simulink model "text28"  (R2014a)
settings: Solver=FixedStepDiscrete  StartTime=0.0  StopTime=10.0  FixedStep=0.0005  RelTol=1e-3
libraries: simulink x70, ec55xxlib x61
(part 2 of 3)

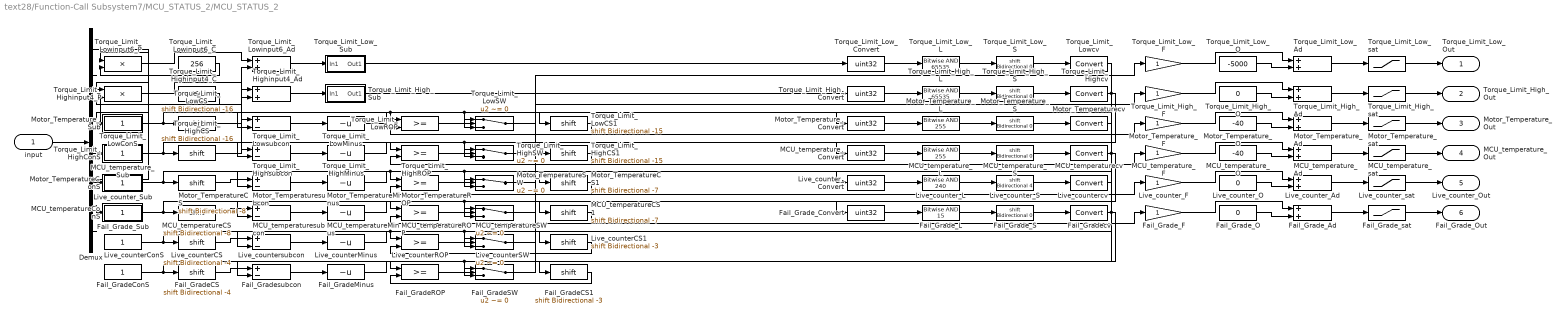
== system text28/Function-Call Subsystem7/MCU_STATUS_2/MCU_STATUS_2 ==
  input : Inport
  Demux : Demux  Outputs=8
  Fail_GradeCS : ArithShift  BitShiftNumber=-4
  Fail_GradeCS1 : ArithShift  BitShiftNumber=-3
  Fail_GradeConS : Constant  OutDataTypeStr=single
  Fail_GradeMinus : UnaryMinus
  Fail_GradeROP : RelationalOperator  OutDataTypeStr=boolean
  Fail_GradeSW : Switch  Criteria=u2 ~= 0
  Fail_Grade_Ad : Sum
  Fail_Grade_Convert : DataTypeConversion  OutDataTypeStr=uint32
  Fail_Grade_F : Gain
  Fail_Grade_L : simulink/Logic and Bit Operations/Bitwise Operator  logicop=AND  UseBitMask=on  BitMask=15  BitMaskRealWorld=Stored Integer
  Fail_Grade_O : Constant  Value=0  OutDataTypeStr=single
  Fail_Grade_S : ArithShift
  Fail_Grade_Sub : Subsystem
  Fail_Grade_sat : Saturate  UpperLimit=4  LowerLimit=0
  Fail_Gradecv : DataTypeConversion
  Fail_Gradesubcon : Sum  Inputs=+-
  Live_counterCS : ArithShift  BitShiftNumber=-4
  Live_counterCS1 : ArithShift  BitShiftNumber=-3
  Live_counterConS : Constant  OutDataTypeStr=single
  Live_counterMinus : UnaryMinus
  Live_counterROP : RelationalOperator  OutDataTypeStr=boolean
  Live_counterSW : Switch  Criteria=u2 ~= 0
  Live_counter_Ad : Sum
  Live_counter_Convert : DataTypeConversion  OutDataTypeStr=uint32
  Live_counter_F : Gain
  Live_counter_L : simulink/Logic and Bit Operations/Bitwise Operator  logicop=AND  UseBitMask=on  BitMask=240  BitMaskRealWorld=Stored Integer
  Live_counter_O : Constant  Value=0  OutDataTypeStr=single
  Live_counter_S : ArithShift  BitShiftNumber=4
  Live_counter_Sub : Subsystem
  Live_counter_sat : Saturate  UpperLimit=15  LowerLimit=0
  Live_countercv : DataTypeConversion
  Live_countersubcon : Sum  Inputs=+-
  MCU_temperatureCS : ArithShift  BitShiftNumber=-8
  MCU_temperatureCS1 : ArithShift  BitShiftNumber=-7
  MCU_temperatureConS : Constant  OutDataTypeStr=single
  MCU_temperatureMinus : UnaryMinus
  MCU_temperatureROP : RelationalOperator  OutDataTypeStr=boolean
  MCU_temperatureSW : Switch  Criteria=u2 ~= 0
  MCU_temperature_Ad : Sum
  MCU_temperature_Convert : DataTypeConversion  OutDataTypeStr=uint32
  MCU_temperature_F : Gain
  MCU_temperature_L : simulink/Logic and Bit Operations/Bitwise Operator  logicop=AND  UseBitMask=on  BitMask=255  BitMaskRealWorld=Stored Integer
  MCU_temperature_O : Constant  Value=-40  OutDataTypeStr=single
  MCU_temperature_S : ArithShift
  MCU_temperature_Sub : Subsystem
  MCU_temperature_sat : Saturate  UpperLimit=215  LowerLimit=-40
  MCU_temperaturecv : DataTypeConversion
  MCU_temperaturesubcon : Sum  Inputs=+-
  Motor_TemperatureCS : ArithShift  BitShiftNumber=-8
  Motor_TemperatureCS1 : ArithShift  BitShiftNumber=-7
  Motor_TemperatureConS : Constant  OutDataTypeStr=single
  Motor_TemperatureMinus : UnaryMinus
  Motor_TemperatureROP : RelationalOperator  OutDataTypeStr=boolean
  Motor_TemperatureSW : Switch  Criteria=u2 ~= 0
  Motor_Temperature_Ad : Sum
  Motor_Temperature_Convert : DataTypeConversion  OutDataTypeStr=uint32
  Motor_Temperature_F : Gain
  Motor_Temperature_L : simulink/Logic and Bit Operations/Bitwise Operator  logicop=AND  UseBitMask=on  BitMask=255  BitMaskRealWorld=Stored Integer
  Motor_Temperature_O : Constant  Value=-40  OutDataTypeStr=single
  Motor_Temperature_S : ArithShift
  Motor_Temperature_Sub : Subsystem
  Motor_Temperature_sat : Saturate  UpperLimit=215  LowerLimit=-40
  Motor_Temperaturecv : DataTypeConversion
  Motor_Temperaturesubcon : Sum  Inputs=+-
  Torque_Limit_HighCS : ArithShift  BitShiftNumber=-16
  Torque_Limit_HighCS1 : ArithShift  BitShiftNumber=-15
  Torque_Limit_HighConS : Constant  OutDataTypeStr=single
  Torque_Limit_HighMinus : UnaryMinus
  Torque_Limit_HighROP : RelationalOperator  OutDataTypeStr=boolean
  Torque_Limit_HighSW : Switch  Criteria=u2 ~= 0
  Torque_Limit_High_Ad : Sum
  Torque_Limit_High_Convert : DataTypeConversion  OutDataTypeStr=uint32
  Torque_Limit_High_F : Gain
  Torque_Limit_High_L : simulink/Logic and Bit Operations/Bitwise Operator  logicop=AND  UseBitMask=on  BitMask=65535  BitMaskRealWorld=Stored Integer
  Torque_Limit_High_O : Constant  Value=0  OutDataTypeStr=single
  Torque_Limit_High_S : ArithShift
  Torque_Limit_High_Sub : Subsystem
  Torque_Limit_High_sat : Saturate  UpperLimit=5000  LowerLimit=0
  Torque_Limit_Highcv : DataTypeConversion
  Torque_Limit_Highinput4_Ad : Sum
  Torque_Limit_Highinput4_C : Constant  Value=256
  Torque_Limit_Highinput4_P : Product
  Torque_Limit_Highsubcon : Sum  Inputs=+-
  Torque_Limit_LowCS : ArithShift  BitShiftNumber=-16
  Torque_Limit_LowCS1 : ArithShift  BitShiftNumber=-15
  Torque_Limit_LowConS : Constant  OutDataTypeStr=single
  Torque_Limit_LowMinus : UnaryMinus
  Torque_Limit_LowROP : RelationalOperator  OutDataTypeStr=boolean
  Torque_Limit_LowSW : Switch  Criteria=u2 ~= 0
  Torque_Limit_Low_Ad : Sum
  Torque_Limit_Low_Convert : DataTypeConversion  OutDataTypeStr=uint32
  Torque_Limit_Low_F : Gain
  Torque_Limit_Low_L : simulink/Logic and Bit Operations/Bitwise Operator  logicop=AND  UseBitMask=on  BitMask=65535  BitMaskRealWorld=Stored Integer
  Torque_Limit_Low_O : Constant  Value=-5000  OutDataTypeStr=single
  Torque_Limit_Low_S : ArithShift
  Torque_Limit_Low_Sub : Subsystem
  Torque_Limit_Low_sat : Saturate  UpperLimit=0  LowerLimit=-5000
  Torque_Limit_Lowcv : DataTypeConversion
  Torque_Limit_Lowinput6_Ad : Sum
  Torque_Limit_Lowinput6_C : Constant  Value=256
  Torque_Limit_Lowinput6_P : Product
  Torque_Limit_Lowsubcon : Sum  Inputs=+-
  Torque_Limit_Low_Out : Outport
  Torque_Limit_High_Out : Outport  Port=2
  Motor_Temperature_Out : Outport  Port=3
  MCU_temperature_Out : Outport  Port=4
  Live_counter_Out : Outport  Port=5
  Fail_Grade_Out : Outport  Port=6
  wires:
  Torque_Limit_Low_F/1 -> Torque_Limit_Low_Ad/1
  Torque_Limit_Low_O/1 -> Torque_Limit_Low_Ad/2
  Torque_Limit_Low_Ad/1 -> Torque_Limit_Low_sat/1
  Torque_Limit_Low_sat/1 -> Torque_Limit_Low_Out/1
  Demux/6 -> Torque_Limit_Lowinput6_P/1
  Torque_Limit_Lowinput6_C/1 -> Torque_Limit_Lowinput6_P/2
  Torque_Limit_Lowinput6_P/1 -> Torque_Limit_Lowinput6_Ad/1
  Demux/5 -> Torque_Limit_Lowinput6_Ad/2
  Torque_Limit_Lowinput6_Ad/1 -> Torque_Limit_Low_Sub/1(In1)
  Torque_Limit_Low_Sub/1(Out1) -> Torque_Limit_Low_Convert/1
  Torque_Limit_Low_Convert/1 -> Torque_Limit_Low_L/1
  Torque_Limit_Low_L/1 -> Torque_Limit_Low_S/1
  Torque_Limit_Low_S/1 -> Torque_Limit_Lowcv/1
  Torque_Limit_Lowcv/1 -> Torque_Limit_LowROP/1, Torque_Limit_Lowsubcon/2, Torque_Limit_LowSW/3
  Torque_Limit_LowConS/1 -> Torque_Limit_LowCS/1, Torque_Limit_LowCS1/1
  Torque_Limit_LowCS1/1 -> Torque_Limit_LowROP/2
  Torque_Limit_LowCS/1 -> Torque_Limit_Lowsubcon/1
  Torque_Limit_Lowsubcon/1 -> Torque_Limit_LowMinus/1
  Torque_Limit_LowMinus/1 -> Torque_Limit_LowSW/1
  Torque_Limit_LowSW/1 -> Torque_Limit_Low_F/1
  Torque_Limit_LowROP/1 -> Torque_Limit_LowSW/2
  Torque_Limit_High_F/1 -> Torque_Limit_High_Ad/1
  Torque_Limit_High_O/1 -> Torque_Limit_High_Ad/2
  Torque_Limit_High_Ad/1 -> Torque_Limit_High_sat/1
  Torque_Limit_High_sat/1 -> Torque_Limit_High_Out/1
  Demux/4 -> Torque_Limit_Highinput4_P/1
  Torque_Limit_Highinput4_C/1 -> Torque_Limit_Highinput4_P/2
  Torque_Limit_Highinput4_P/1 -> Torque_Limit_Highinput4_Ad/1
  Demux/3 -> Torque_Limit_Highinput4_Ad/2
  Torque_Limit_Highinput4_Ad/1 -> Torque_Limit_High_Sub/1(In1)
  Torque_Limit_High_Sub/1(Out1) -> Torque_Limit_High_Convert/1
  Torque_Limit_High_Convert/1 -> Torque_Limit_High_L/1
  Torque_Limit_High_L/1 -> Torque_Limit_High_S/1
  Torque_Limit_High_S/1 -> Torque_Limit_Highcv/1
  Torque_Limit_Highcv/1 -> Torque_Limit_Highsubcon/2, Torque_Limit_HighSW/3, Torque_Limit_HighROP/1
  Torque_Limit_HighConS/1 -> Torque_Limit_HighCS/1, Torque_Limit_HighCS1/1
  Torque_Limit_HighCS1/1 -> Torque_Limit_HighROP/2
  Torque_Limit_HighCS/1 -> Torque_Limit_Highsubcon/1
  Torque_Limit_Highsubcon/1 -> Torque_Limit_HighMinus/1
  Torque_Limit_HighMinus/1 -> Torque_Limit_HighSW/1
  Torque_Limit_HighSW/1 -> Torque_Limit_High_F/1
  Torque_Limit_HighROP/1 -> Torque_Limit_HighSW/2
  Motor_Temperature_F/1 -> Motor_Temperature_Ad/1
  Motor_Temperature_O/1 -> Motor_Temperature_Ad/2
  Motor_Temperature_Ad/1 -> Motor_Temperature_sat/1
  Motor_Temperature_sat/1 -> Motor_Temperature_Out/1
  Demux/1 -> Motor_Temperature_Sub/1(In1)
  Motor_Temperature_Sub/1(Out1) -> Motor_Temperature_Convert/1
  Motor_Temperature_Convert/1 -> Motor_Temperature_L/1
  Motor_Temperature_L/1 -> Motor_Temperature_S/1
  Motor_Temperature_S/1 -> Motor_Temperaturecv/1
  Motor_Temperaturecv/1 -> Motor_TemperatureROP/1, Motor_Temperaturesubcon/2, Motor_TemperatureSW/3
  Motor_TemperatureConS/1 -> Motor_TemperatureCS/1, Motor_TemperatureCS1/1
  Motor_TemperatureCS1/1 -> Motor_TemperatureROP/2
  Motor_TemperatureCS/1 -> Motor_Temperaturesubcon/1
  Motor_Temperaturesubcon/1 -> Motor_TemperatureMinus/1
  Motor_TemperatureMinus/1 -> Motor_TemperatureSW/1
  Motor_TemperatureSW/1 -> Motor_Temperature_F/1
  Motor_TemperatureROP/1 -> Motor_TemperatureSW/2
  MCU_temperature_F/1 -> MCU_temperature_Ad/1
  MCU_temperature_O/1 -> MCU_temperature_Ad/2
  MCU_temperature_Ad/1 -> MCU_temperature_sat/1
  MCU_temperature_sat/1 -> MCU_temperature_Out/1
  Demux/2 -> MCU_temperature_Sub/1(In1)
  MCU_temperature_Sub/1(Out1) -> MCU_temperature_Convert/1
  MCU_temperature_Convert/1 -> MCU_temperature_L/1
  MCU_temperature_L/1 -> MCU_temperature_S/1
  MCU_temperature_S/1 -> MCU_temperaturecv/1
  MCU_temperaturecv/1 -> MCU_temperaturesubcon/2, MCU_temperatureSW/3, MCU_temperatureROP/1
  MCU_temperatureConS/1 -> MCU_temperatureCS/1, MCU_temperatureCS1/1
  MCU_temperatureCS1/1 -> MCU_temperatureROP/2
  MCU_temperatureCS/1 -> MCU_temperaturesubcon/1
  MCU_temperaturesubcon/1 -> MCU_temperatureMinus/1
  MCU_temperatureMinus/1 -> MCU_temperatureSW/1
  MCU_temperatureSW/1 -> MCU_temperature_F/1
  MCU_temperatureROP/1 -> MCU_temperatureSW/2
  Live_counter_F/1 -> Live_counter_Ad/1
  Live_counter_O/1 -> Live_counter_Ad/2
  Live_counter_Ad/1 -> Live_counter_sat/1
  Live_counter_sat/1 -> Live_counter_Out/1
  Demux/8 -> Live_counter_Sub/1(In1)
  Live_counter_Sub/1(Out1) -> Live_counter_Convert/1
  Live_counter_Convert/1 -> Live_counter_L/1
  Live_counter_L/1 -> Live_counter_S/1
  Live_counter_S/1 -> Live_countercv/1
  Live_countercv/1 -> Live_counterROP/1, Live_countersubcon/2, Live_counterSW/3
  Live_counterConS/1 -> Live_counterCS/1, Live_counterCS1/1
  Live_counterCS1/1 -> Live_counterROP/2
  Live_counterCS/1 -> Live_countersubcon/1
  Live_countersubcon/1 -> Live_counterMinus/1
  Live_counterMinus/1 -> Live_counterSW/1
  Live_counterSW/1 -> Live_counter_F/1
  Live_counterROP/1 -> Live_counterSW/2
  Fail_Grade_F/1 -> Fail_Grade_Ad/1
  Fail_Grade_O/1 -> Fail_Grade_Ad/2
  Fail_Grade_Ad/1 -> Fail_Grade_sat/1
  Fail_Grade_sat/1 -> Fail_Grade_Out/1
  Demux/7 -> Fail_Grade_Sub/1(In1)
  Fail_Grade_Sub/1(Out1) -> Fail_Grade_Convert/1
  Fail_Grade_Convert/1 -> Fail_Grade_L/1
  Fail_Grade_L/1 -> Fail_Grade_S/1
  Fail_Grade_S/1 -> Fail_Gradecv/1
  Fail_Gradecv/1 -> Fail_Gradesubcon/2, Fail_GradeSW/3, Fail_GradeROP/1
  Fail_GradeConS/1 -> Fail_GradeCS/1, Fail_GradeCS1/1
  Fail_GradeCS1/1 -> Fail_GradeROP/2
  Fail_GradeCS/1 -> Fail_Gradesubcon/1
  Fail_Gradesubcon/1 -> Fail_GradeMinus/1
  Fail_GradeMinus/1 -> Fail_GradeSW/1
  Fail_GradeSW/1 -> Fail_Grade_F/1
  Fail_GradeROP/1 -> Fail_GradeSW/2
  input/1 -> Demux/1

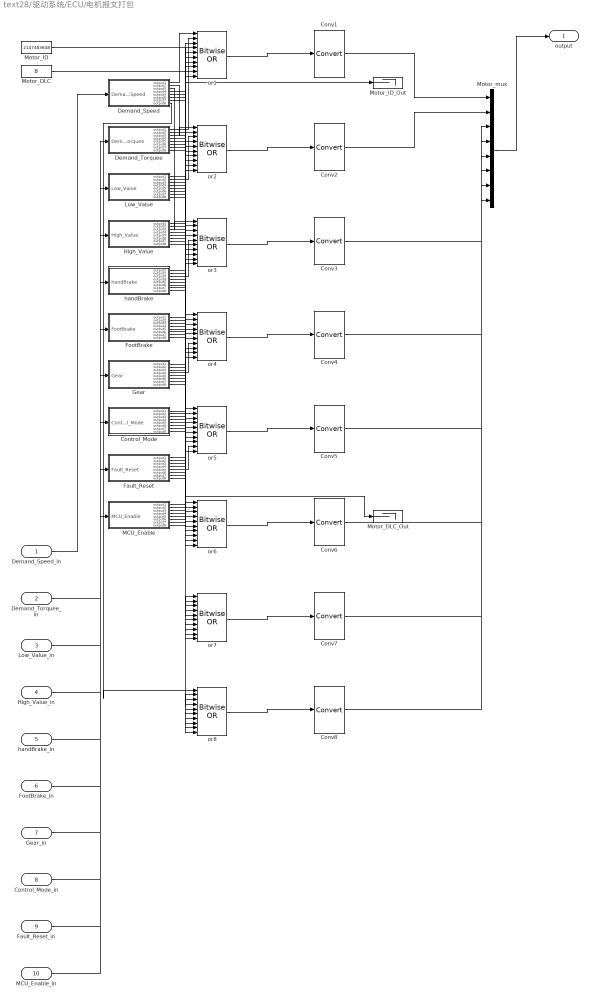
== system text28/驱动系统/ECU/电机报文打包 ==
  Demand_Speed_in : Inport
  Demand_Torquee_in : Inport  Port=2
  Low_Value_in : Inport  Port=3
  High_Value_in : Inport  Port=4
  handBrake_in : Inport  Port=5
  FootBrake_in : Inport  Port=6
  Gear_in : Inport  Port=7
  Control_Mode_in : Inport  Port=8
  Fault_Reset_in : Inport  Port=9
  MCU_Enable_in : Inport  Port=10
  Control_Mode : Subsystem
  Conv{1..8} (8 alike) : DataTypeConversion
  Demand_Speed : Subsystem
  Demand_Torquee : Subsystem
  Fault_Reset : Subsystem
  FootBrake : Subsystem
  Gear : Subsystem
  High_Value : Subsystem
  Low_Value : Subsystem
  MCU_Enable : Subsystem
  Motor_DLC : Constant  Value=8  OutDataTypeStr=uint8
  Motor_DLC_Out : Terminator
  Motor_ID : Constant  Value=2147483648  OutDataTypeStr=single
  Motor_ID_Out : Terminator
  Motor_mux : Mux  Inputs=8
  handBrake : Subsystem
  or{1..8} (8 alike) : simulink/Logic and Bit Operations/Bitwise Operator  logicop=OR  UseBitMask=off  NumInputPorts=10  BitMask=bin2dec('11011001')  BitMaskRealWorld=Stored Integer
  output : Outport
  wires:
  MCU_Enable_in/1 -> MCU_Enable/1(MCU_Enable)
  Fault_Reset_in/1 -> Fault_Reset/1(Fault_Reset)
  Control_Mode_in/1 -> Control_Mode/1(Control_Mode)
  Gear_in/1 -> Gear/1(Gear)
  FootBrake_in/1 -> FootBrake/1(FootBrake)
  handBrake_in/1 -> handBrake/1(handBrake)
  High_Value_in/1 -> High_Value/1(High_Value)
  Low_Value_in/1 -> Low_Value/1(Low_Value)
  Demand_Torquee_in/1 -> Demand_Torquee/1(Demand_Torquee)
  Demand_Speed_in/1 -> Demand_Speed/1(Demand_Speed)
  Motor_DLC/1 -> Motor_DLC_Out/1
  Motor_ID/1 -> Motor_ID_Out/1
  Conv8/1 -> Motor_mux/8
  or8/1 -> Conv8/1
  Conv7/1 -> Motor_mux/7
  or7/1 -> Conv7/1
  Conv6/1 -> Motor_mux/6
  or6/1 -> Conv6/1
  Conv5/1 -> Motor_mux/5
  or5/1 -> Conv5/1
  Conv4/1 -> Motor_mux/4
  or4/1 -> Conv4/1
  Conv3/1 -> Motor_mux/3
  or3/1 -> Conv3/1
  Conv2/1 -> Motor_mux/2
  or2/1 -> Conv2/1
  Conv1/1 -> Motor_mux/1
  or1/1 -> Conv1/1
  MCU_Enable/8(output8) -> or8/10
  MCU_Enable/7(output7) -> or7/10
  MCU_Enable/6(output6) -> or6/10
  MCU_Enable/5(output5) -> or5/10
  MCU_Enable/4(output4) -> or4/10
  MCU_Enable/3(output3) -> or3/10
  MCU_Enable/2(output2) -> or2/10
  MCU_Enable/1(output1) -> or1/10
  Fault_Reset/8(output8) -> or8/9
  Fault_Reset/7(output7) -> or7/9
  Fault_Reset/6(output6) -> or6/9
  Fault_Reset/5(output5) -> or5/9
  Fault_Reset/4(output4) -> or4/9
  Fault_Reset/3(output3) -> or3/9
  Fault_Reset/2(output2) -> or2/9
  Fault_Reset/1(output1) -> or1/9
  Control_Mode/8(output8) -> or8/8
  Control_Mode/7(output7) -> or7/8
  Control_Mode/6(output6) -> or6/8
  Control_Mode/5(output5) -> or5/8
  Control_Mode/4(output4) -> or4/8
  Control_Mode/3(output3) -> or3/8
  Control_Mode/2(output2) -> or2/8
  Control_Mode/1(output1) -> or1/8
  Gear/8(output8) -> or8/7
  Gear/7(output7) -> or7/7
  Gear/6(output6) -> or6/7
  Gear/5(output5) -> or5/7
  Gear/4(output4) -> or4/7
  Gear/3(output3) -> or3/7
  Gear/2(output2) -> or2/7
  Gear/1(output1) -> or1/7
  FootBrake/8(output8) -> or8/6
  FootBrake/7(output7) -> or7/6
  FootBrake/6(output6) -> or6/6
  FootBrake/5(output5) -> or5/6
  FootBrake/4(output4) -> or4/6
  FootBrake/3(output3) -> or3/6
  FootBrake/2(output2) -> or2/6
  FootBrake/1(output1) -> or1/6
  handBrake/8(output8) -> or8/5
  handBrake/7(output7) -> or7/5
  handBrake/6(output6) -> or6/5
  handBrake/5(output5) -> or5/5
  handBrake/4(output4) -> or4/5
  handBrake/3(output3) -> or3/5
  handBrake/2(output2) -> or2/5
  handBrake/1(output1) -> or1/5
  High_Value/8(output8) -> or8/4
  High_Value/7(output7) -> or7/4
  High_Value/6(output6) -> or6/4
  High_Value/5(output5) -> or5/4
  High_Value/4(output4) -> or4/4
  High_Value/3(output3) -> or3/4
  High_Value/2(output2) -> or2/4
  High_Value/1(output1) -> or1/4
  Low_Value/8(output8) -> or8/3
  Low_Value/7(output7) -> or7/3
  Low_Value/6(output6) -> or6/3
  Low_Value/5(output5) -> or5/3
  Low_Value/4(output4) -> or4/3
  Low_Value/3(output3) -> or3/3
  Low_Value/2(output2) -> or2/3
  Low_Value/1(output1) -> or1/3
  Demand_Torquee/8(output8) -> or8/2
  Demand_Torquee/7(output7) -> or7/2
  Demand_Torquee/6(output6) -> or6/2
  Demand_Torquee/5(output5) -> or5/2
  Demand_Torquee/4(output4) -> or4/2
  Demand_Torquee/3(output3) -> or3/2
  Demand_Torquee/2(output2) -> or2/2
  Demand_Torquee/1(output1) -> or1/2
  Demand_Speed/8(output8) -> or8/1
  Demand_Speed/7(output7) -> or7/1
  Demand_Speed/6(output6) -> or6/1
  Demand_Speed/5(output5) -> or5/1
  Demand_Speed/4(output4) -> or4/1
  Demand_Speed/3(output3) -> or3/1
  Demand_Speed/2(output2) -> or2/1
  Demand_Speed/1(output1) -> or1/1
  Motor_mux/1 -> output/1

== system text28/驱动系统/MCU_CAN发送/安全回路out ==
  CAN ok : Inport
  Data Type Conversion1 : DataTypeConversion  OutDataTypeStr=double
  If : If  IfExpression=u1 < 2
  If Action Subsystem1 : Subsystem  TreatAsAtomicUnit=on
  If Action Subsystem2 : Subsystem  TreatAsAtomicUnit=on
  Merge : Merge
  Out1 : Outport
  wires:
  If/1 -> If Action Subsystem2/Action
  If/2 -> If Action Subsystem1/Action
  If Action Subsystem1/1(Out2) -> Merge/2
  If Action Subsystem2/1(Out1) -> Merge/1
  CAN ok/1 -> Data Type Conversion1/1
  Data Type Conversion1/1 -> If/1
  Merge/1 -> Out1/1

== system text28/驱动系统/驱动逻辑/Drive_AEKF ==
  T_base : Inport
  w_rpm : Inport  Port=2
  Te_raw : Inport  Port=3
  T_base_d : DataTypeConversion  OutDataTypeStr=double  SaturateOnIntegerOverflow=on  RndMeth=Zero
  Te_raw_d : DataTypeConversion  OutDataTypeStr=double  SaturateOnIntegerOverflow=on  RndMeth=Zero
  TorqueDelta : Sum  Inputs=+-  SaturateOnIntegerOverflow=on  InputSameDT=on  OutDataTypeStr=Inherit: Same as first input
  TorqueDeltaSat : Saturate  UpperLimit=25  LowerLimit=-50
  TorquePrev : UnitDelay  SampleTime=-1
  TorqueSum : Sum  SaturateOnIntegerOverflow=on  InputSameDT=on  OutDataTypeStr=Inherit: Same as first input
  aekf_comp : MATLAB Function  TreatAsAtomicUnit=on
  w_rpm_d : DataTypeConversion  OutDataTypeStr=double  SaturateOnIntegerOverflow=on  RndMeth=Zero
  T_opt : Outport
  wires:
  T_base/1 -> T_base_d/1
  w_rpm/1 -> w_rpm_d/1
  Te_raw/1 -> Te_raw_d/1
  T_base_d/1 -> aekf_comp/1(T_base)
  w_rpm_d/1 -> aekf_comp/2(w_rpm)
  Te_raw_d/1 -> aekf_comp/3(Te_raw)
  aekf_comp/1(T_opt) -> TorqueDelta/1
  TorquePrev/1 -> TorqueDelta/2, TorqueSum/1
  TorqueDelta/1 -> TorqueDeltaSat/1
  TorqueDeltaSat/1 -> TorqueSum/2
  TorqueSum/1 -> T_opt/1, TorquePrev/1

== system text28/驱动系统/驱动逻辑/制动与尾灯 ==
  Constant2 : Constant  OutDataTypeStr=uint32  SampleTime=-1
  Data Type Conversion : DataTypeConversion  OutDataTypeStr=uint32
  If : If  IfExpression=u1 > 550 &u1 < 4600
  If Action Subsystem : Subsystem  TreatAsAtomicUnit=on
  If Action Subsystem1 : Subsystem  TreatAsAtomicUnit=on
  If Action Subsystem2 : Subsystem  TreatAsAtomicUnit=on
  If Action Subsystem3 : Subsystem  TreatAsAtomicUnit=on
  If1 : If  IfExpression=u1 > 850 &u1 < 4600
  MeaModule : ec55xxlib/RapidECU_U2/11Calibration/MeaModule  signal=youya1
  MeaModule1 : ec55xxlib/RapidECU_U2/11Calibration/MeaModule  signal=youya2
  MeaModule2 : ec55xxlib/RapidECU_U2/11Calibration/MeaModule  signal=youya3
  Merge1 : Merge
  Merge4 : Merge
  前油压 : ec55xxlib/RapidECU_U2/02AnalogInput/AnalogInput  channel=54: I_AN15_5V  sampletime=-1
  尾灯 : ec55xxlib/RapidECU_U2/06PowerDriverPWM/PowerDriverPWM  channel=115: O_PWM10_HS2A9  sampletime=-1
  油压2 : Outport
  油压1 : Outport  Port=2
  wires:
  If/1 -> If Action Subsystem/Action
  If/2 -> If Action Subsystem1/Action
  If Action Subsystem1/1(Out1) -> Merge4/2
  If Action Subsystem/1(Out1) -> Merge4/1
  Constant2/1 -> 尾灯/1
  Data Type Conversion/1 -> 尾灯/2
  前油压/1 -> MeaModule/1
  Merge4/1 -> MeaModule1/1, Data Type Conversion/1
  If1/1 -> If Action Subsystem2/Action
  If1/2 -> If Action Subsystem3/Action
  If Action Subsystem3/1(Out1) -> Merge1/2
  If Action Subsystem2/1(Out1) -> Merge1/1
  MeaModule/1 -> If1/1, If/1
  Merge1/1 -> MeaModule2/1
  MeaModule2/1 -> 油压2/1
  MeaModule1/1 -> 油压1/1

== system text28/驱动系统/驱动逻辑/制动与待驶 ==
  note: `
  "制动 " : Inport
  Constant : Constant  Value=0  SampleTime=-1
  Constant1 : Constant  SampleTime=-1
  Logical Operator : Logic  AllPortsSameDT=off  OutDataTypeStr=boolean
  MeaModule : ec55xxlib/RapidECU_U2/11Calibration/MeaModule  signal=enable_sign
  MeaModule1 : ec55xxlib/RapidECU_U2/11Calibration/MeaModule  signal=daishi
  MeaModule2 : ec55xxlib/RapidECU_U2/11Calibration/MeaModule  signal=aqhl
  MeaModule3 : ec55xxlib/RapidECU_U2/11Calibration/MeaModule  signal=daishi_chu
  MeaModule4 : ec55xxlib/RapidECU_U2/11Calibration/MeaModule  signal=daishi_fanhui
  MeaModule5 : ec55xxlib/RapidECU_U2/11Calibration/MeaModule  signal=daishi_out
  Product : Product
  Saturation : Saturate  UpperLimit=1  LowerLimit=0
  Sum : Sum  Inputs=|++
  Switch : Switch  Criteria=u2 > Threshold
  SwitchInput : ec55xxlib/RapidECU_U2/01SwitchInput/SwitchInput  channel=44: I_SW11_H  sampletime=-1
  Unit Delay : UnitDelay  SampleTime=-1
  待驶按键 : Subsystem
  待驶激活 : Subsystem
  鸣笛1 : Subsystem
  RES : Outport
  EN : Outport  Port=2
  wires:
  Constant/1 -> Switch/1
  Constant1/1 -> Switch/3
  Switch/1 -> RES/1
  Saturation/1 -> MeaModule/1
  Unit Delay/1 -> MeaModule4/1
  "制动 "/1 -> 待驶激活/1(制动)
  待驶激活/1(Out1) -> MeaModule5/1
  MeaModule/1 -> Switch/2, 鸣笛1/1("鸣笛 "), EN/1
  待驶按键/1(待驶in) -> MeaModule1/1
  MeaModule1/1 -> 待驶激活/2(按钮)
  Sum/1 -> MeaModule3/1
  SwitchInput/1 -> MeaModule2/1
  MeaModule2/1 -> 鸣笛1/2("安全回路 "), Product/1
  MeaModule4/1 -> Sum/2
  MeaModule5/1 -> Sum/1
  Product/1 -> Unit Delay/1, Saturation/1
  MeaModule3/1 -> Product/2

== system text28/驱动系统/驱动逻辑/油门规则 ==
  油门原始值 : Inport
  油门百分比 : Inport  Port=2
  刹车有效 : Inport  Port=3
  MeaModule : ec55xxlib/RapidECU_U2/11Calibration/MeaModule  signal=apps_rule
  MeaModule1 : ec55xxlib/RapidECU_U2/11Calibration/MeaModule  signal=zuizhong
  Product : Product
  Product1 : Product
  Sum : Sum
  Unit Delay : UnitDelay  InitialCondition=1  SampleTime=-1
  刹车判断 : Subsystem
  动力允许判断 : Subsystem
  油门刹车冲突 : Subsystem
  油门死区判断 : Subsystem
  油门请求 : Outport
  wires:
  油门百分比/1 -> 油门死区判断/1(In1), 油门刹车冲突/1(油门)
  油门刹车冲突/1(Out1) -> Sum/2
  Unit Delay/1 -> 油门刹车冲突/3(反馈)
  动力允许判断/1(Out1) -> Unit Delay/1, MeaModule/1
  Sum/1 -> 动力允许判断/1(In1)
  Product/1 -> Sum/1
  刹车判断/1(Out1) -> Product/2
  油门死区判断/1(Out1) -> Product/1
  MeaModule/1 -> Product1/2
  Product1/1 -> MeaModule1/1
  MeaModule1/1 -> 油门请求/1
  油门原始值/1 -> Product1/1
  刹车有效/1 -> 刹车判断/1(In1), 油门刹车冲突/2(刹车)

== system text28/驱动系统/驱动逻辑/电机测速 ==
  CANReceive : ec55xxlib/RapidECU_U2/07CANCommucation/CANReceive  canmodule=B  canbuffer=7  canmessageid=hex2dec('CFF0009')  canmessagetype=Extended(29-bit ID)  datalength=8  sampletime=-1
  Function-Call Subsystem4 : Subsystem  TreatAsAtomicUnit=on
  ReceiveMessages : Subsystem
  电机转速 : Outport
  电机扭矩 : Outport  Port=2
  wires:
  Function-Call Subsystem4/1("Out2 ") -> ReceiveMessages/1(resive)
  CANReceive/2 -> Function-Call Subsystem4/1(In3)
  CANReceive/5 -> Function-Call Subsystem4/4(In4)
  CANReceive/4 -> Function-Call Subsystem4/3(In2)
  CANReceive/1 -> Function-Call Subsystem4/Trigger
  CANReceive/3 -> Function-Call Subsystem4/2(In1)
  ReceiveMessages/1(电机转速) -> 电机转速/1
  ReceiveMessages/2(电机扭矩) -> 电机扭矩/1

== system text28/驱动系统/驱动逻辑/角度传感器 ==
  MeaModule : ec55xxlib/RapidECU_U2/11Calibration/MeaModule  signal=app_date2
  MeaModule1 : ec55xxlib/RapidECU_U2/11Calibration/MeaModule  signal=jiaodu_2222
  MeaModule2 : ec55xxlib/RapidECU_U2/11Calibration/MeaModule  signal=jiaodu_11111
  MeaModule4 : ec55xxlib/RapidECU_U2/11Calibration/MeaModule  signal=app_scs
  角度1 : ec55xxlib/RapidECU_U2/02AnalogInput/AnalogInput  channel=52: I_AN13_5V  sampletime=-1
  角度2 : ec55xxlib/RapidECU_U2/02AnalogInput/AnalogInput  channel=53: I_AN14_5V  sampletime=-1
  角度传感器数据处理及不可靠信号 : Subsystem  TreatAsAtomicUnit=on
  角度传感器是否正常 : Subsystem
  "油门数值 " : Outport
  油门百分比 : Outport  Port=2
  系统关键信号判断 : Outport  Port=3
  wires:
  角度传感器是否正常/1(油门范围) -> MeaModule4/1
  MeaModule4/1 -> 系统关键信号判断/1
  角度2/1 -> MeaModule1/1
  角度1/1 -> MeaModule2/1, 角度传感器是否正常/1(角度1)
  角度传感器数据处理及不可靠信号/1(油门数值) -> MeaModule/1
  MeaModule/1 -> "油门数值 "/1
  角度传感器数据处理及不可靠信号/2(油门百分比) -> 油门百分比/1
  MeaModule2/1 -> 角度传感器数据处理及不可靠信号/1(角度1)
  MeaModule1/1 -> 角度传感器数据处理及不可靠信号/2(角度2), 角度传感器是否正常/2(角度2)

== system text28/Function-Call Subsystem4/ReceiveMessages/BMS_HCU_INFO/BatAlmLv_Sub ==
  In1 : Inport
  Out1 : Outport
  wires:
  In1/1 -> Out1/1

== system text28/Function-Call Subsystem4/ReceiveMessages/BMS_HCU_INFO/BatCurrent_Sub ==
  In1 : Inport
  Out1 : Outport
  wires:
  In1/1 -> Out1/1

== system text28/Function-Call Subsystem4/ReceiveMessages/BMS_HCU_INFO/BatLife_Sub ==
  In1 : Inport
  Out1 : Outport
  wires:
  In1/1 -> Out1/1

== system text28/Function-Call Subsystem4/ReceiveMessages/BMS_HCU_INFO/BatSoc_Sub ==
  In1 : Inport
  Out1 : Outport
  wires:
  In1/1 -> Out1/1

== system text28/Function-Call Subsystem4/ReceiveMessages/BMS_HCU_INFO/BatState_Sub ==
  In1 : Inport
  Out1 : Outport
  wires:
  In1/1 -> Out1/1

== system text28/Function-Call Subsystem4/ReceiveMessages/BMS_HCU_INFO/BatVoltage_Sub ==
  In1 : Inport
  Out1 : Outport
  wires:
  In1/1 -> Out1/1

== system text28/Function-Call Subsystem4/ReceiveMessages/BMS_HCU_INFO/BtaSOH_Sub ==
  In1 : Inport
  Out1 : Outport
  wires:
  In1/1 -> Out1/1

== system text28/Function-Call Subsystem7/MCU_STATUS_2/MCU_STATUS_2/Fail_Grade_Sub ==
  In1 : Inport
  Out1 : Outport
  wires:
  In1/1 -> Out1/1

== system text28/Function-Call Subsystem7/MCU_STATUS_2/MCU_STATUS_2/Live_counter_Sub ==
  In1 : Inport
  Out1 : Outport
  wires:
  In1/1 -> Out1/1

== system text28/Function-Call Subsystem7/MCU_STATUS_2/MCU_STATUS_2/MCU_temperature_Sub ==
  In1 : Inport
  Out1 : Outport
  wires:
  In1/1 -> Out1/1

== system text28/Function-Call Subsystem7/MCU_STATUS_2/MCU_STATUS_2/Motor_Temperature_Sub ==
  In1 : Inport
  Out1 : Outport
  wires:
  In1/1 -> Out1/1

== system text28/Function-Call Subsystem7/MCU_STATUS_2/MCU_STATUS_2/Torque_Limit_High_Sub ==
  In1 : Inport
  Out1 : Outport
  wires:
  In1/1 -> Out1/1

== system text28/Function-Call Subsystem7/MCU_STATUS_2/MCU_STATUS_2/Torque_Limit_Low_Sub ==
  In1 : Inport
  Out1 : Outport
  wires:
  In1/1 -> Out1/1

== system text28/驱动系统/ECU/电机报文打包/Control_Mode ==
  Control_Mode : Inport
  Constant{2..8} (7 alike) : Constant  Value=0  OutDataTypeStr=uint8  SampleTime=-1
  Control_ModeRon : Rounding  Operator=round
  Control_Mode_1sat : Saturate  UpperLimit=12  LowerLimit=0
  Control_Mode_Convert : DataTypeConversion  OutDataTypeStr=uint8
  Control_Mode_Convert1 : DataTypeConversion  OutDataTypeStr=uint32
  Control_Mode_D : Product  Inputs=*/
  Control_Mode_F : Constant  OutDataTypeStr=single
  Control_Mode_L : simulink/Logic and Bit Operations/Bitwise Operator  logicop=AND  UseBitMask=on  BitMask=12  BitMaskRealWorld=Stored Integer
  Control_Mode_O : Constant  Value=0  OutDataTypeStr=single
  Control_Mode_S : ArithShift  BitShiftNumber=-2
  Control_Mode_sat : Saturate  UpperLimit=2  LowerLimit=0
  Control_Mode_st : Sum  Inputs=+-
  output1 : Outport
  output2 : Outport  Port=2
  output3 : Outport  Port=3
  output4 : Outport  Port=4
  output5 : Outport  Port=5
  output6 : Outport  Port=6
  output7 : Outport  Port=7
  output8 : Outport  Port=8
  wires:
  Constant8/1 -> output8/1
  Constant7/1 -> output7/1
  Constant6/1 -> output6/1
  Constant5/1 -> output5/1
  Constant4/1 -> output4/1
  Constant3/1 -> output3/1
  Constant2/1 -> output2/1
  Control_Mode_Convert/1 -> output1/1
  Control_Mode_L/1 -> Control_Mode_Convert/1
  Control_Mode_Convert1/1 -> Control_Mode_L/1
  Control_Mode_1sat/1 -> Control_Mode_Convert1/1
  Control_Mode_S/1 -> Control_Mode_1sat/1
  Control_ModeRon/1 -> Control_Mode_S/1
  Control_Mode_D/1 -> Control_ModeRon/1
  Control_Mode_F/1 -> Control_Mode_D/2
  Control_Mode_st/1 -> Control_Mode_D/1
  Control_Mode_O/1 -> Control_Mode_st/2
  Control_Mode_sat/1 -> Control_Mode_st/1
  Control_Mode/1 -> Control_Mode_sat/1

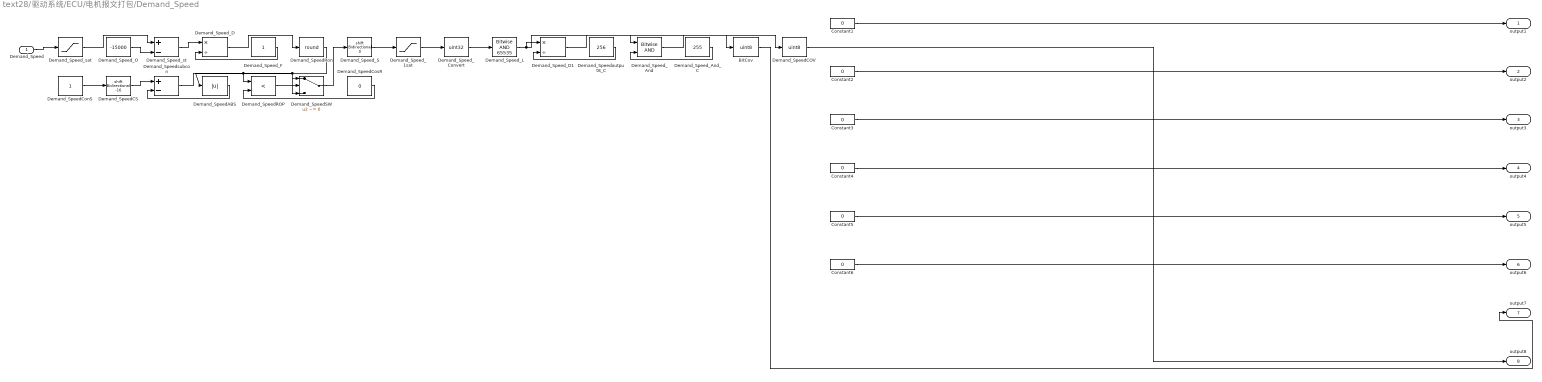
== system text28/驱动系统/ECU/电机报文打包/Demand_Speed ==
  Demand_Speed : Inport
  BitCov : DataTypeConversion  OutDataTypeStr=uint8
  Constant{1..6} (6 alike) : Constant  Value=0  OutDataTypeStr=uint8  SampleTime=-1
  Demand_SpeedABS : Abs
  Demand_SpeedCOV : DataTypeConversion  OutDataTypeStr=uint8
  Demand_SpeedCS : ArithShift  BitShiftNumber=-16
  Demand_SpeedConS : Constant  OutDataTypeStr=single
  Demand_SpeedCosR : Constant  Value=0  OutDataTypeStr=uint8
  Demand_SpeedROP : RelationalOperator  Operator=<  OutDataTypeStr=boolean
  Demand_SpeedRon : Rounding  Operator=round
  Demand_SpeedSW : Switch  Criteria=u2 ~= 0
  Demand_Speed_1sat : Saturate  UpperLimit=65535  LowerLimit=0
  Demand_Speed_And : simulink/Logic and Bit Operations/Bitwise Operator  logicop=AND  UseBitMask=off  NumInputPorts=2  BitMask=bin2dec('11011001')  BitMaskRealWorld=Stored Integer
  Demand_Speed_And_C : Constant  Value=255  OutDataTypeStr=uint32
  Demand_Speed_Convert : DataTypeConversion  OutDataTypeStr=uint32
  Demand_Speed_D : Product  Inputs=*/
  Demand_Speed_D1 : Product  Inputs=*/
  Demand_Speed_F : Constant  OutDataTypeStr=single
  Demand_Speed_L : simulink/Logic and Bit Operations/Bitwise Operator  logicop=AND  UseBitMask=on  BitMask=65535  BitMaskRealWorld=Stored Integer
  Demand_Speed_O : Constant  Value=-15000  OutDataTypeStr=single
  Demand_Speed_S : ArithShift
  Demand_Speed_sat : Saturate  UpperLimit=15000  LowerLimit=-15000
  Demand_Speed_st : Sum  Inputs=+-
  Demand_Speedoutput8_C : Constant  Value=256
  Demand_Speedsubcon : Sum  Inputs=+-
  output1 : Outport
  output2 : Outport  Port=2
  output3 : Outport  Port=3
  output4 : Outport  Port=4
  output5 : Outport  Port=5
  output6 : Outport  Port=6
  output7 : Outport  Port=7
  output8 : Outport  Port=8
  wires:
  Constant6/1 -> output6/1
  Constant5/1 -> output5/1
  Constant4/1 -> output4/1
  Constant3/1 -> output3/1
  Constant2/1 -> output2/1
  Constant1/1 -> output1/1
  BitCov/1 -> output7/1
  Demand_Speed_And/1 -> BitCov/1
  Demand_Speed_And_C/1 -> Demand_Speed_And/2
  Demand_SpeedCOV/1 -> output8/1
  Demand_Speed_D1/1 -> Demand_SpeedCOV/1
  Demand_Speedoutput8_C/1 -> Demand_Speed_D1/2
  Demand_Speed_L/1 -> Demand_Speed_And/1, Demand_Speed_D1/1
  Demand_Speed_Convert/1 -> Demand_Speed_L/1
  Demand_Speed_1sat/1 -> Demand_Speed_Convert/1
  Demand_Speed_S/1 -> Demand_Speed_1sat/1
  Demand_SpeedSW/1 -> Demand_Speed_S/1
  Demand_SpeedROP/1 -> Demand_SpeedSW/2
  Demand_Speedsubcon/1 -> Demand_SpeedSW/1
  Demand_SpeedABS/1 -> Demand_Speedsubcon/2
  Demand_SpeedCS/1 -> Demand_Speedsubcon/1
  Demand_SpeedConS/1 -> Demand_SpeedCS/1
  Demand_SpeedCosR/1 -> Demand_SpeedROP/2
  Demand_SpeedRon/1 -> Demand_SpeedABS/1, Demand_SpeedROP/1, Demand_SpeedSW/3
  Demand_Speed_D/1 -> Demand_SpeedRon/1
  Demand_Speed_F/1 -> Demand_Speed_D/2
  Demand_Speed_st/1 -> Demand_Speed_D/1
  Demand_Speed_O/1 -> Demand_Speed_st/2
  Demand_Speed_sat/1 -> Demand_Speed_st/1
  Demand_Speed/1 -> Demand_Speed_sat/1

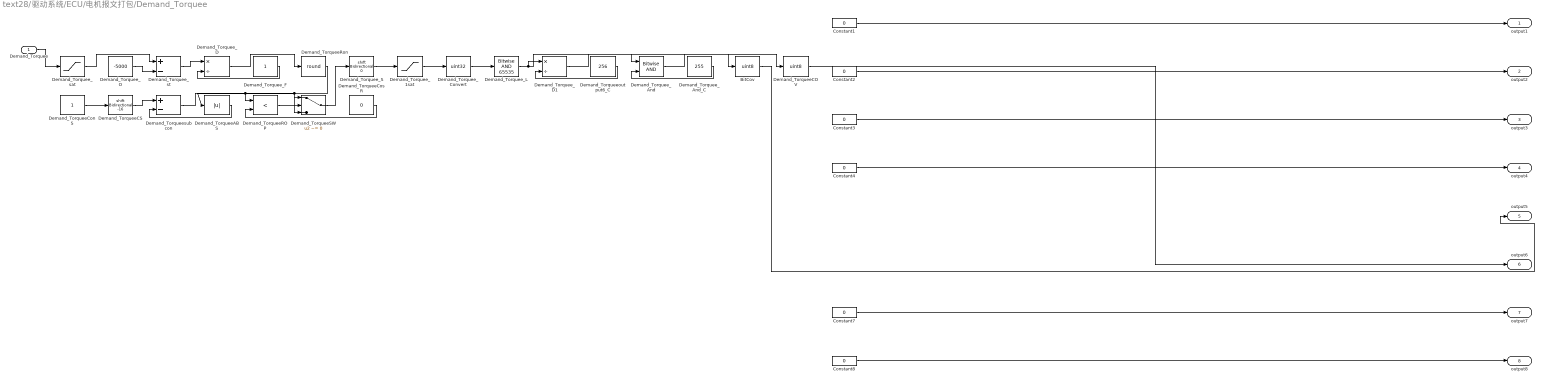
== system text28/驱动系统/ECU/电机报文打包/Demand_Torquee ==
  Demand_Torquee : Inport
  BitCov : DataTypeConversion  OutDataTypeStr=uint8
  Constant{1..4,7..8} (6 alike) : Constant  Value=0  OutDataTypeStr=uint8  SampleTime=-1
  Demand_TorqueeABS : Abs
  Demand_TorqueeCOV : DataTypeConversion  OutDataTypeStr=uint8
  Demand_TorqueeCS : ArithShift  BitShiftNumber=-16
  Demand_TorqueeConS : Constant  OutDataTypeStr=single
  Demand_TorqueeCosR : Constant  Value=0  OutDataTypeStr=uint8
  Demand_TorqueeROP : RelationalOperator  Operator=<  OutDataTypeStr=boolean
  Demand_TorqueeRon : Rounding  Operator=round
  Demand_TorqueeSW : Switch  Criteria=u2 ~= 0
  Demand_Torquee_1sat : Saturate  UpperLimit=65535  LowerLimit=0
  Demand_Torquee_And : simulink/Logic and Bit Operations/Bitwise Operator  logicop=AND  UseBitMask=off  NumInputPorts=2  BitMask=bin2dec('11011001')  BitMaskRealWorld=Stored Integer
  Demand_Torquee_And_C : Constant  Value=255  OutDataTypeStr=uint32
  Demand_Torquee_Convert : DataTypeConversion  OutDataTypeStr=uint32
  Demand_Torquee_D : Product  Inputs=*/
  Demand_Torquee_D1 : Product  Inputs=*/
  Demand_Torquee_F : Constant  OutDataTypeStr=single
  Demand_Torquee_L : simulink/Logic and Bit Operations/Bitwise Operator  logicop=AND  UseBitMask=on  BitMask=65535  BitMaskRealWorld=Stored Integer
  Demand_Torquee_O : Constant  Value=-5000  OutDataTypeStr=single
  Demand_Torquee_S : ArithShift
  Demand_Torquee_sat : Saturate  UpperLimit=5000  LowerLimit=-5000
  Demand_Torquee_st : Sum  Inputs=+-
  Demand_Torqueeoutput6_C : Constant  Value=256
  Demand_Torqueesubcon : Sum  Inputs=+-
  output1 : Outport
  output2 : Outport  Port=2
  output3 : Outport  Port=3
  output4 : Outport  Port=4
  output5 : Outport  Port=5
  output6 : Outport  Port=6
  output7 : Outport  Port=7
  output8 : Outport  Port=8
  wires:
  Constant8/1 -> output8/1
  Constant7/1 -> output7/1
  Constant4/1 -> output4/1
  Constant3/1 -> output3/1
  Constant2/1 -> output2/1
  Constant1/1 -> output1/1
  BitCov/1 -> output5/1
  Demand_Torquee_And/1 -> BitCov/1
  Demand_Torquee_And_C/1 -> Demand_Torquee_And/2
  Demand_TorqueeCOV/1 -> output6/1
  Demand_Torquee_D1/1 -> Demand_TorqueeCOV/1
  Demand_Torqueeoutput6_C/1 -> Demand_Torquee_D1/2
  Demand_Torquee_L/1 -> Demand_Torquee_And/1, Demand_Torquee_D1/1
  Demand_Torquee_Convert/1 -> Demand_Torquee_L/1
  Demand_Torquee_1sat/1 -> Demand_Torquee_Convert/1
  Demand_Torquee_S/1 -> Demand_Torquee_1sat/1
  Demand_TorqueeSW/1 -> Demand_Torquee_S/1
  Demand_TorqueeROP/1 -> Demand_TorqueeSW/2
  Demand_Torqueesubcon/1 -> Demand_TorqueeSW/1
  Demand_TorqueeABS/1 -> Demand_Torqueesubcon/2
  Demand_TorqueeCS/1 -> Demand_Torqueesubcon/1
  Demand_TorqueeConS/1 -> Demand_TorqueeCS/1
  Demand_TorqueeCosR/1 -> Demand_TorqueeROP/2
  Demand_TorqueeRon/1 -> Demand_TorqueeSW/3, Demand_TorqueeABS/1, Demand_TorqueeROP/1
  Demand_Torquee_D/1 -> Demand_TorqueeRon/1
  Demand_Torquee_F/1 -> Demand_Torquee_D/2
  Demand_Torquee_st/1 -> Demand_Torquee_D/1
  Demand_Torquee_O/1 -> Demand_Torquee_st/2
  Demand_Torquee_sat/1 -> Demand_Torquee_st/1
  Demand_Torquee/1 -> Demand_Torquee_sat/1

== system text28/驱动系统/ECU/电机报文打包/Fault_Reset ==
  Fault_Reset : Inport
  Constant{2..8} (7 alike) : Constant  Value=0  OutDataTypeStr=uint8  SampleTime=-1
  Fault_ResetRon : Rounding  Operator=round
  Fault_Reset_1sat : Saturate  UpperLimit=2  LowerLimit=0
  Fault_Reset_Convert : DataTypeConversion  OutDataTypeStr=uint8
  Fault_Reset_Convert1 : DataTypeConversion  OutDataTypeStr=uint32
  Fault_Reset_D : Product  Inputs=*/
  Fault_Reset_F : Constant  OutDataTypeStr=single
  Fault_Reset_L : simulink/Logic and Bit Operations/Bitwise Operator  logicop=AND  UseBitMask=on  BitMask=2  BitMaskRealWorld=Stored Integer
  Fault_Reset_O : Constant  Value=0  OutDataTypeStr=single
  Fault_Reset_S : ArithShift  BitShiftNumber=-1
  Fault_Reset_sat : Saturate  UpperLimit=1  LowerLimit=0
  Fault_Reset_st : Sum  Inputs=+-
  output1 : Outport
  output2 : Outport  Port=2
  output3 : Outport  Port=3
  output4 : Outport  Port=4
  output5 : Outport  Port=5
  output6 : Outport  Port=6
  output7 : Outport  Port=7
  output8 : Outport  Port=8
  wires:
  Constant8/1 -> output8/1
  Constant7/1 -> output7/1
  Constant6/1 -> output6/1
  Constant5/1 -> output5/1
  Constant4/1 -> output4/1
  Constant3/1 -> output3/1
  Constant2/1 -> output2/1
  Fault_Reset_Convert/1 -> output1/1
  Fault_Reset_L/1 -> Fault_Reset_Convert/1
  Fault_Reset_Convert1/1 -> Fault_Reset_L/1
  Fault_Reset_1sat/1 -> Fault_Reset_Convert1/1
  Fault_Reset_S/1 -> Fault_Reset_1sat/1
  Fault_ResetRon/1 -> Fault_Reset_S/1
  Fault_Reset_D/1 -> Fault_ResetRon/1
  Fault_Reset_F/1 -> Fault_Reset_D/2
  Fault_Reset_st/1 -> Fault_Reset_D/1
  Fault_Reset_O/1 -> Fault_Reset_st/2
  Fault_Reset_sat/1 -> Fault_Reset_st/1
  Fault_Reset/1 -> Fault_Reset_sat/1

== system text28/驱动系统/ECU/电机报文打包/FootBrake ==
  FootBrake : Inport
  Constant{2..8} (7 alike) : Constant  Value=0  OutDataTypeStr=uint8  SampleTime=-1
  FootBrakeRon : Rounding  Operator=round
  FootBrake_1sat : Saturate  UpperLimit=64  LowerLimit=0
  FootBrake_Convert : DataTypeConversion  OutDataTypeStr=uint8
  FootBrake_Convert1 : DataTypeConversion  OutDataTypeStr=uint32
  FootBrake_D : Product  Inputs=*/
  FootBrake_F : Constant  OutDataTypeStr=single
  FootBrake_L : simulink/Logic and Bit Operations/Bitwise Operator  logicop=AND  UseBitMask=on  BitMask=64  BitMaskRealWorld=Stored Integer
  FootBrake_O : Constant  Value=0  OutDataTypeStr=single
  FootBrake_S : ArithShift  BitShiftNumber=-6
  FootBrake_sat : Saturate  UpperLimit=1  LowerLimit=0
  FootBrake_st : Sum  Inputs=+-
  output1 : Outport
  output2 : Outport  Port=2
  output3 : Outport  Port=3
  output4 : Outport  Port=4
  output5 : Outport  Port=5
  output6 : Outport  Port=6
  output7 : Outport  Port=7
  output8 : Outport  Port=8
  wires:
  Constant8/1 -> output8/1
  Constant7/1 -> output7/1
  Constant6/1 -> output6/1
  Constant5/1 -> output5/1
  Constant4/1 -> output4/1
  Constant3/1 -> output3/1
  Constant2/1 -> output2/1
  FootBrake_Convert/1 -> output1/1
  FootBrake_L/1 -> FootBrake_Convert/1
  FootBrake_Convert1/1 -> FootBrake_L/1
  FootBrake_1sat/1 -> FootBrake_Convert1/1
  FootBrake_S/1 -> FootBrake_1sat/1
  FootBrakeRon/1 -> FootBrake_S/1
  FootBrake_D/1 -> FootBrakeRon/1
  FootBrake_F/1 -> FootBrake_D/2
  FootBrake_st/1 -> FootBrake_D/1
  FootBrake_O/1 -> FootBrake_st/2
  FootBrake_sat/1 -> FootBrake_st/1
  FootBrake/1 -> FootBrake_sat/1

== system text28/驱动系统/ECU/电机报文打包/Gear ==
  Gear : Inport
  Constant{2..8} (7 alike) : Constant  Value=0  OutDataTypeStr=uint8  SampleTime=-1
  GearRon : Rounding  Operator=round
  Gear_1sat : Saturate  UpperLimit=48  LowerLimit=0
  Gear_Convert : DataTypeConversion  OutDataTypeStr=uint8
  Gear_Convert1 : DataTypeConversion  OutDataTypeStr=uint32
  Gear_D : Product  Inputs=*/
  Gear_F : Constant  OutDataTypeStr=single
  Gear_L : simulink/Logic and Bit Operations/Bitwise Operator  logicop=AND  UseBitMask=on  BitMask=48  BitMaskRealWorld=Stored Integer
  Gear_O : Constant  Value=0  OutDataTypeStr=single
  Gear_S : ArithShift  BitShiftNumber=-4
  Gear_sat : Saturate  UpperLimit=2  LowerLimit=0
  Gear_st : Sum  Inputs=+-
  output1 : Outport
  output2 : Outport  Port=2
  output3 : Outport  Port=3
  output4 : Outport  Port=4
  output5 : Outport  Port=5
  output6 : Outport  Port=6
  output7 : Outport  Port=7
  output8 : Outport  Port=8
  wires:
  Constant8/1 -> output8/1
  Constant7/1 -> output7/1
  Constant6/1 -> output6/1
  Constant5/1 -> output5/1
  Constant4/1 -> output4/1
  Constant3/1 -> output3/1
  Constant2/1 -> output2/1
  Gear_Convert/1 -> output1/1
  Gear_L/1 -> Gear_Convert/1
  Gear_Convert1/1 -> Gear_L/1
  Gear_1sat/1 -> Gear_Convert1/1
  Gear_S/1 -> Gear_1sat/1
  GearRon/1 -> Gear_S/1
  Gear_D/1 -> GearRon/1
  Gear_F/1 -> Gear_D/2
  Gear_st/1 -> Gear_D/1
  Gear_O/1 -> Gear_st/2
  Gear_sat/1 -> Gear_st/1
  Gear/1 -> Gear_sat/1

== system text28/驱动系统/ECU/电机报文打包/High_Value ==
  High_Value : Inport
  Constant{1,4..8} (6 alike) : Constant  Value=0  OutDataTypeStr=uint8  SampleTime=-1
  High_ValueBitCov : DataTypeConversion  OutDataTypeStr=uint8
  High_ValueCOV : DataTypeConversion  OutDataTypeStr=uint8
  High_ValueRon : Rounding  Operator=round
  High_Value_1sat : Saturate  UpperLimit=4095  LowerLimit=0
  High_Value_And : simulink/Logic and Bit Operations/Bitwise Operator  logicop=AND  UseBitMask=off  NumInputPorts=2  BitMask=bin2dec('11011001')  BitMaskRealWorld=Stored Integer
  High_Value_And_C : Constant  Value=255  OutDataTypeStr=uint32
  High_Value_Convert : DataTypeConversion  OutDataTypeStr=uint32
  High_Value_D : Product  Inputs=*/
  High_Value_D1 : Product  Inputs=*/
  High_Value_F : Constant  Value=4  OutDataTypeStr=single
  High_Value_L : simulink/Logic and Bit Operations/Bitwise Operator  logicop=AND  UseBitMask=on  BitMask=4095  BitMaskRealWorld=Stored Integer
  High_Value_O : Constant  Value=0  OutDataTypeStr=single
  High_Value_S : ArithShift
  High_Value_sat : Saturate  UpperLimit=16384  LowerLimit=0
  High_Value_st : Sum  Inputs=+-
  High_Valueoutput3_C : Constant  Value=256
  output1 : Outport
  output2 : Outport  Port=2
  output3 : Outport  Port=3
  output4 : Outport  Port=4
  output5 : Outport  Port=5
  output6 : Outport  Port=6
  output7 : Outport  Port=7
  output8 : Outport  Port=8
  wires:
  Constant8/1 -> output8/1
  Constant7/1 -> output7/1
  Constant6/1 -> output6/1
  Constant5/1 -> output5/1
  Constant4/1 -> output4/1
  Constant1/1 -> output1/1
  High_ValueBitCov/1 -> output2/1
  High_Value_And/1 -> High_ValueBitCov/1
  High_Value_And_C/1 -> High_Value_And/2
  High_ValueCOV/1 -> output3/1
  High_Value_D1/1 -> High_ValueCOV/1
  High_Valueoutput3_C/1 -> High_Value_D1/2
  High_Value_L/1 -> High_Value_And/1, High_Value_D1/1
  High_Value_Convert/1 -> High_Value_L/1
  High_Value_1sat/1 -> High_Value_Convert/1
  High_Value_S/1 -> High_Value_1sat/1
  High_ValueRon/1 -> High_Value_S/1
  High_Value_D/1 -> High_ValueRon/1
  High_Value_F/1 -> High_Value_D/2
  High_Value_st/1 -> High_Value_D/1
  High_Value_O/1 -> High_Value_st/2
  High_Value_sat/1 -> High_Value_st/1
  High_Value/1 -> High_Value_sat/1

== system text28/驱动系统/ECU/电机报文打包/Low_Value ==
  Low_Value : Inport
  Constant{1..2,5..8} (6 alike) : Constant  Value=0  OutDataTypeStr=uint8  SampleTime=-1
  Low_ValueBitCov : DataTypeConversion  OutDataTypeStr=uint8
  Low_ValueCOV : DataTypeConversion  OutDataTypeStr=uint8
  Low_ValueRon : Rounding  Operator=round
  Low_Value_1sat : Saturate  UpperLimit=65520  LowerLimit=0
  Low_Value_And : simulink/Logic and Bit Operations/Bitwise Operator  logicop=AND  UseBitMask=off  NumInputPorts=2  BitMask=bin2dec('11011001')  BitMaskRealWorld=Stored Integer
  Low_Value_And_C : Constant  Value=255  OutDataTypeStr=uint32
  Low_Value_Convert : DataTypeConversion  OutDataTypeStr=uint32
  Low_Value_D : Product  Inputs=*/
  Low_Value_D1 : Product  Inputs=*/
  Low_Value_F : Constant  Value=4  OutDataTypeStr=single
  Low_Value_L : simulink/Logic and Bit Operations/Bitwise Operator  logicop=AND  UseBitMask=on  BitMask=65520  BitMaskRealWorld=Stored Integer
  Low_Value_O : Constant  Value=0  OutDataTypeStr=single
  Low_Value_S : ArithShift  BitShiftNumber=-4
  Low_Value_sat : Saturate  UpperLimit=16384  LowerLimit=0
  Low_Value_st : Sum  Inputs=+-
  Low_Valueoutput4_C : Constant  Value=256
  output1 : Outport
  output2 : Outport  Port=2
  output3 : Outport  Port=3
  output4 : Outport  Port=4
  output5 : Outport  Port=5
  output6 : Outport  Port=6
  output7 : Outport  Port=7
  output8 : Outport  Port=8
  wires:
  Constant8/1 -> output8/1
  Constant7/1 -> output7/1
  Constant6/1 -> output6/1
  Constant5/1 -> output5/1
  Constant2/1 -> output2/1
  Constant1/1 -> output1/1
  Low_ValueBitCov/1 -> output3/1
  Low_Value_And/1 -> Low_ValueBitCov/1
  Low_Value_And_C/1 -> Low_Value_And/2
  Low_ValueCOV/1 -> output4/1
  Low_Value_D1/1 -> Low_ValueCOV/1
  Low_Valueoutput4_C/1 -> Low_Value_D1/2
  Low_Value_L/1 -> Low_Value_And/1, Low_Value_D1/1
  Low_Value_Convert/1 -> Low_Value_L/1
  Low_Value_1sat/1 -> Low_Value_Convert/1
  Low_Value_S/1 -> Low_Value_1sat/1
  Low_ValueRon/1 -> Low_Value_S/1
  Low_Value_D/1 -> Low_ValueRon/1
  Low_Value_F/1 -> Low_Value_D/2
  Low_Value_st/1 -> Low_Value_D/1
  Low_Value_O/1 -> Low_Value_st/2
  Low_Value_sat/1 -> Low_Value_st/1
  Low_Value/1 -> Low_Value_sat/1

== system text28/驱动系统/ECU/电机报文打包/MCU_Enable ==
  MCU_Enable : Inport
  Constant{2..8} (7 alike) : Constant  Value=0  OutDataTypeStr=uint8  SampleTime=-1
  MCU_EnableRon : Rounding  Operator=round
  MCU_Enable_1sat : Saturate  UpperLimit=1  LowerLimit=0
  MCU_Enable_Convert : DataTypeConversion  OutDataTypeStr=uint8
  MCU_Enable_Convert1 : DataTypeConversion  OutDataTypeStr=uint32
  MCU_Enable_D : Product  Inputs=*/
  MCU_Enable_F : Constant  OutDataTypeStr=single
  MCU_Enable_L : simulink/Logic and Bit Operations/Bitwise Operator  logicop=AND  UseBitMask=on  BitMask=1  BitMaskRealWorld=Stored Integer
  MCU_Enable_O : Constant  Value=0  OutDataTypeStr=single
  MCU_Enable_S : ArithShift
  MCU_Enable_sat : Saturate  UpperLimit=1  LowerLimit=0
  MCU_Enable_st : Sum  Inputs=+-
  output1 : Outport
  output2 : Outport  Port=2
  output3 : Outport  Port=3
  output4 : Outport  Port=4
  output5 : Outport  Port=5
  output6 : Outport  Port=6
  output7 : Outport  Port=7
  output8 : Outport  Port=8
  wires:
  Constant8/1 -> output8/1
  Constant7/1 -> output7/1
  Constant6/1 -> output6/1
  Constant5/1 -> output5/1
  Constant4/1 -> output4/1
  Constant3/1 -> output3/1
  Constant2/1 -> output2/1
  MCU_Enable_Convert/1 -> output1/1
  MCU_Enable_L/1 -> MCU_Enable_Convert/1
  MCU_Enable_Convert1/1 -> MCU_Enable_L/1
  MCU_Enable_1sat/1 -> MCU_Enable_Convert1/1
  MCU_Enable_S/1 -> MCU_Enable_1sat/1
  MCU_EnableRon/1 -> MCU_Enable_S/1
  MCU_Enable_D/1 -> MCU_EnableRon/1
  MCU_Enable_F/1 -> MCU_Enable_D/2
  MCU_Enable_st/1 -> MCU_Enable_D/1
  MCU_Enable_O/1 -> MCU_Enable_st/2
  MCU_Enable_sat/1 -> MCU_Enable_st/1
  MCU_Enable/1 -> MCU_Enable_sat/1

== system text28/驱动系统/ECU/电机报文打包/handBrake ==
  handBrake : Inport
  Constant{2..8} (7 alike) : Constant  Value=0  OutDataTypeStr=uint8  SampleTime=-1
  handBrakeRon : Rounding  Operator=round
  handBrake_1sat : Saturate  UpperLimit=128  LowerLimit=0
  handBrake_Convert : DataTypeConversion  OutDataTypeStr=uint8
  handBrake_Convert1 : DataTypeConversion  OutDataTypeStr=uint32
  handBrake_D : Product  Inputs=*/
  handBrake_F : Constant  OutDataTypeStr=single
  handBrake_L : simulink/Logic and Bit Operations/Bitwise Operator  logicop=AND  UseBitMask=on  BitMask=128  BitMaskRealWorld=Stored Integer
  handBrake_O : Constant  Value=0  OutDataTypeStr=single
  handBrake_S : ArithShift  BitShiftNumber=-7
  handBrake_sat : Saturate  UpperLimit=0  LowerLimit=0
  handBrake_st : Sum  Inputs=+-
  output1 : Outport
  output2 : Outport  Port=2
  output3 : Outport  Port=3
  output4 : Outport  Port=4
  output5 : Outport  Port=5
  output6 : Outport  Port=6
  output7 : Outport  Port=7
  output8 : Outport  Port=8
  wires:
  Constant8/1 -> output8/1
  Constant7/1 -> output7/1
  Constant6/1 -> output6/1
  Constant5/1 -> output5/1
  Constant4/1 -> output4/1
  Constant3/1 -> output3/1
  Constant2/1 -> output2/1
  handBrake_Convert/1 -> output1/1
  handBrake_L/1 -> handBrake_Convert/1
  handBrake_Convert1/1 -> handBrake_L/1
  handBrake_1sat/1 -> handBrake_Convert1/1
  handBrake_S/1 -> handBrake_1sat/1
  handBrakeRon/1 -> handBrake_S/1
  handBrake_D/1 -> handBrakeRon/1
  handBrake_F/1 -> handBrake_D/2
  handBrake_st/1 -> handBrake_D/1
  handBrake_O/1 -> handBrake_st/2
  handBrake_sat/1 -> handBrake_st/1
  handBrake/1 -> handBrake_sat/1

== system text28/驱动系统/MCU_CAN发送/安全回路out/If Action Subsystem1 ==
  Action Port : ActionPort  ActionType=else
  Constant1 : Constant  Value=0  OutDataTypeStr=uint32
  Data Type Conversion2 : DataTypeConversion  OutDataTypeStr=double
  Out2 : Outport
  wires:
  Constant1/1 -> Data Type Conversion2/1
  Data Type Conversion2/1 -> Out2/1

== system text28/驱动系统/MCU_CAN发送/安全回路out/If Action Subsystem2 ==
  Action Port : ActionPort  ActionType=then
  Constant : Constant
  Out1 : Outport
  wires:
  Constant/1 -> Out1/1

== system text28/驱动系统/驱动逻辑/制动与尾灯/If Action Subsystem ==
  Action Port : ActionPort  ActionType=then
  Constant : Constant  SampleTime=-1
  Out1 : Outport
  wires:
  Constant/1 -> Out1/1

== system text28/驱动系统/驱动逻辑/制动与尾灯/If Action Subsystem1 ==
  Action Port : ActionPort  ActionType=else
  Constant : Constant  Value=0  SampleTime=-1
  Out1 : Outport
  wires:
  Constant/1 -> Out1/1

== system text28/驱动系统/驱动逻辑/制动与尾灯/If Action Subsystem2 ==
  Action Port : ActionPort  ActionType=then
  Constant : Constant  SampleTime=-1
  Out1 : Outport
  wires:
  Constant/1 -> Out1/1

== system text28/驱动系统/驱动逻辑/制动与尾灯/If Action Subsystem3 ==
  Action Port : ActionPort  ActionType=else
  Constant : Constant  Value=0  SampleTime=-1
  Out1 : Outport
  wires:
  Constant/1 -> Out1/1

== system text28/驱动系统/驱动逻辑/制动与待驶/待驶按键 ==
  Constant : Constant  SampleTime=-1
  Constant1 : Constant  Value=0  SampleTime=-1
  MeaModule3 : ec55xxlib/RapidECU_U2/11Calibration/MeaModule  signal=daishi_11
  PowerDriverSwitchDiagnosis : ec55xxlib/RapidECU_U2/06PowerDriverPWM/PowerDriverSwitchDiagnosis  channel=82: O_PWM5_LS1A8  sampletime=-1
  Switch : Switch  Criteria=u2 > Threshold
  待驶in : Outport
  wires:
  Constant/1 -> Switch/3
  Constant1/1 -> Switch/1
  PowerDriverSwitchDiagnosis/1 -> MeaModule3/1
  MeaModule3/1 -> Switch/2
  Switch/1 -> 待驶in/1

== system text28/驱动系统/驱动逻辑/制动与待驶/待驶激活 ==
  制动 : Inport
  按钮 : Inport  Port=2
  If : If
  If Action Subsystem : Subsystem  TreatAsAtomicUnit=on
  If Action Subsystem1 : Subsystem  TreatAsAtomicUnit=on
  If Action Subsystem2 : Subsystem  TreatAsAtomicUnit=on
  If Action Subsystem3 : Subsystem  TreatAsAtomicUnit=on
  If1 : If
  Logical Operator : Logic  AllPortsSameDT=off  OutDataTypeStr=boolean
  Merge : Merge
  Merge1 : Merge
  Out1 : Outport
  wires:
  If/1 -> If Action Subsystem/Action
  If/2 -> If Action Subsystem1/Action
  If1/1 -> If Action Subsystem2/Action
  If1/2 -> If Action Subsystem3/Action
  按钮/1 -> If/1
  制动/1 -> If1/1
  Logical Operator/1 -> Out1/1
  If Action Subsystem/1(Out1) -> Merge/1
  If Action Subsystem1/1(Out1) -> Merge/2
  If Action Subsystem2/1(Out1) -> Merge1/1
  If Action Subsystem3/1(Out1) -> Merge1/2
  Merge/1 -> Logical Operator/1
  Merge1/1 -> Logical Operator/2

== system text28/驱动系统/驱动逻辑/制动与待驶/鸣笛1 ==
  "鸣笛 " : Inport
  "安全回路 " : Inport  Port=2
  If : If
  If Action Subsystem : Subsystem  TreatAsAtomicUnit=on
  If Action Subsystem1 : Subsystem  TreatAsAtomicUnit=on
  Merge : Merge
  鸣笛 : Subsystem
  wires:
  If/1 -> If Action Subsystem/Action
  If/2 -> If Action Subsystem1/Action
  If Action Subsystem/1(Out1) -> Merge/1
  If Action Subsystem1/1(Out1) -> Merge/2
  Merge/1 -> 鸣笛/1(In1)
  "鸣笛 "/1 -> If/1
  "安全回路 "/1 -> 鸣笛/2(安全回路)

== system text28/驱动系统/驱动逻辑/油门规则/刹车判断 ==
  In1 : Inport
  If2 : If  IfExpression=u1==0
  Merge1 : Merge
  有刹车 : Subsystem  TreatAsAtomicUnit=on
  没刹车 : Subsystem  TreatAsAtomicUnit=on
  Out1 : Outport
  wires:
  If2/1 -> 没刹车/Action
  If2/2 -> 有刹车/Action
  没刹车/1(Out1) -> Merge1/1
  有刹车/1(Out1) -> Merge1/2
  Merge1/1 -> Out1/1
  In1/1 -> If2/1

== system text28/驱动系统/驱动逻辑/油门规则/动力允许判断 ==
  In1 : Inport
  If3 : If  IfExpression=u1 >=1
  Merge3 : Merge
  动力信号 : Subsystem  TreatAsAtomicUnit=on
  故障信号 : Subsystem  TreatAsAtomicUnit=on
  Out1 : Outport
  wires:
  If3/1 -> 动力信号/Action
  If3/2 -> 故障信号/Action
  In1/1 -> If3/1
  故障信号/1(Out1) -> Merge3/2
  Merge3/1 -> Out1/1
  动力信号/1(Out1) -> Merge3/1
